simulink model "EnabledGenerator_Model"  (R2023a)
settings: Solver=VariableStepAuto  StartTime=0.0  StopTime=10.0  RelTol=1e-3
libraries: NSA_DEVS_SOURCES_ATOMIC x2, NSA_DEVS_SINKS_ATOMIC x2, NSA_DEVS_LOGISTICS_ATOMIC x1
settings Model: Creator=david  LastModifiedBy=david

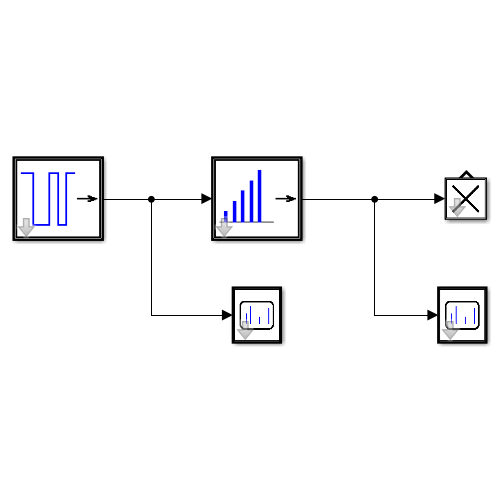
[thumbnail: Simulink's stored preview of the top-level diagram]
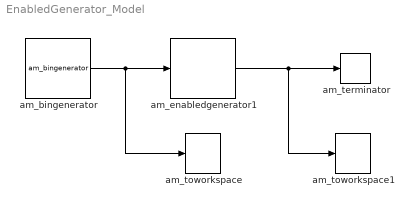
== system EnabledGenerator_Model ==
  am_bingenerator : NSA_DEVS_SOURCES_ATOMIC/am_bingenerator  z0="\"1\""  tVec=[3.0, 6.0, 12, 14, 100]  tau=[0,1]  debug=0
      settings: SourceProductName=NSA_DEVS
  am_enabledgenerator1 : NSA_DEVS_SOURCES_ATOMIC/am_enabledgenerator  tG=0.9  n0=2  nG=11  tau=[0,1]  debug=0
      settings: SourceProductName=NSA_DEVS
  am_terminator : NSA_DEVS_LOGISTICS_ATOMIC/am_terminator  tau=[0,1]  debug=0
      settings: SourceProductName=NSA_DEVS
  am_toworkspace : NSA_DEVS_SINKS_ATOMIC/am_toworkspace  varname="\"bingenOut\""  t0=0  format="\"vector\""  tau=[0,3]  debug=0
      settings: SourceProductName=NSA_DEVS
  am_toworkspace1 : NSA_DEVS_SINKS_ATOMIC/am_toworkspace  varname="\"genOut\""  t0=0  format="\"vector\""  tau=[0,3]  debug=0
      settings: SourceProductName=NSA_DEVS
  wires:
  am_bingenerator/1 -> am_enabledgenerator1/1, am_toworkspace/1
  am_enabledgenerator1/1 -> am_toworkspace1/1, am_terminator/1
